simulink model "Gas_Exchange"  (Simulink 7.0)
settings: Solver=ode45  StartTime=0.0  StopTime=10.0  RelTol=1e-3
values from neighbouring files (symbols this model uses):
  a1 = 0.3836    [Dissociation_Spencer_IC.m]    (also in Gas_Exchange_IC.m; Respiratory_IC.m)
  a2 = 1.819    [Dissociation_Spencer_IC.m]    (also in Gas_Exchange_IC.m; Respiratory_IC.m)
  alpha1 = 0.02598    [Dissociation_Spencer_IC.m]    (also in Gas_Exchange_IC.m; Respiratory_IC.m)
  alpha2 = 0.05591    [Dissociation_Spencer_IC.m]    (also in Gas_Exchange_IC.m; Respiratory_IC.m)
  beta1 = 0.012275    [Dissociation_Spencer_IC.m]    (also in Gas_Exchange_IC.m; Respiratory_IC.m)
  beta2 = 0.03255    [Dissociation_Spencer_IC.m]    (also in Gas_Exchange_IC.m; Respiratory_IC.m)
  C1 = 9    [Dissociation_Spencer_IC.m]    (also in Gas_Exchange_IC.m; Respiratory_IC.m)
  C2 = 87.00    (= 87)    [Dissociation_Spencer_IC.m]    (also in Gas_Exchange_IC.m; Respiratory_IC.m)
  CvCO2IC = 0.5116    [Body_Khoo_IC.m]    (also in Gas_Exchange_IC.m; Respiratory_IC.m = 0.5247)
  CvO2IC = 0.1672    [Body_Khoo_IC.m]    (also in Gas_Exchange_IC.m; Respiratory_IC.m = 0.1639)
  Dead1CO2IC = 0.1020    (= 0.102)    [Dead_Space_Khoo_IC.m]    (also in Gas_Exchange_IC.m; Respiratory_IC.m = 39.5616)
  Dead1O2IC = 149.8824    [Dead_Space_Khoo_IC.m]    (also in Gas_Exchange_IC.m; Respiratory_IC.m = 104.3637)
  Dead2CO2IC = 0.5274    [Dead_Space_Khoo_IC.m]    (also in Gas_Exchange_IC.m; Respiratory_IC.m = 39.6736)
  Dead2O2IC = 149.3923    [Dead_Space_Khoo_IC.m]    (also in Gas_Exchange_IC.m; Respiratory_IC.m = 104.2258)
  Dead3CO2IC = 2.2996    [Dead_Space_Khoo_IC.m]    (also in Gas_Exchange_IC.m; Respiratory_IC.m = 39.8127)
  Dead3O2IC = 147.3503    [Dead_Space_Khoo_IC.m]    (also in Gas_Exchange_IC.m; Respiratory_IC.m = 104.0505)
  Dead4CO2IC = 8.2293    [Dead_Space_Khoo_IC.m]    (also in Gas_Exchange_IC.m; Respiratory_IC.m = 40.0061)
  Dead4O2IC = 140.5179    [Dead_Space_Khoo_IC.m]    (also in Gas_Exchange_IC.m; Respiratory_IC.m = 103.8005)
  Dead5CO2IC = 22.0757    [Dead_Space_Khoo_IC.m]    (also in Gas_Exchange_IC.m; Respiratory_IC.m = 40.3359)
  Dead5O2IC = 124.5641    [Dead_Space_Khoo_IC.m]    (also in Gas_Exchange_IC.m; Respiratory_IC.m = 103.3579)
  h = 0.0183    [Brain_Khoo_IC.m]    (also in Gas_Exchange_IC.m; Respiratory_IC.m)
  K1 = 13    [Dissociation_Spencer_IC.m]    (also in Gas_Exchange_IC.m; Respiratory_IC.m)
  K2 = 194.4    [Dissociation_Spencer_IC.m]    (also in Gas_Exchange_IC.m; Respiratory_IC.m)
  MRbCO2 = 0.0517    [Brain_Khoo_IC.m]    (also in Gas_Exchange_IC.m; Respiratory_IC.m)
  MRCO2 = 0.0033    [Body_Khoo_IC.m]    (also in Gas_Exchange_IC.m; Respiratory_IC.m)
  MRO2 = 0.0038    [Body_Khoo_IC.m]    (also in Gas_Exchange_IC.m; Respiratory_IC.m)
  PACO2_delayIC = 39.6041    [Cardio_Mix_Lange_IC.m]    (also in Gas_Exchange_IC.m; Respiratory_IC.m = 40.4448)
  PaCO2firstIC = 0.2150    (= 0.215)    [Cardio_Mix_Lange_IC.m]    (also in Gas_Exchange_IC.m; Respiratory_IC.m = -0.2465)
  PACO2IC = 37.1484    [Gas_Exchange_IC.m]    (also in Lungs_Khoo_IC.m; Respiratory_IC.m = 40.9432)
  PaCO2secondIC = 38.4577    [Cardio_Mix_Lange_IC.m]    (also in Gas_Exchange_IC.m; Respiratory_IC.m = 40.3928)
  PAO2_delayIC = 103.8436    [Cardio_Mix_Lange_IC.m]    (also in Gas_Exchange_IC.m; Respiratory_IC.m = 103.1223)
  PaO2firstIC = -0.2838    [Cardio_Mix_Lange_IC.m]    (also in Gas_Exchange_IC.m; Respiratory_IC.m = 0.3557)
  PAO2IC = 107.1983    [Gas_Exchange_IC.m]    (also in Lungs_Khoo_IC.m; Respiratory_IC.m = 102.5153)
  PaO2secondIC = 105.4828    [Cardio_Mix_Lange_IC.m]    (also in Gas_Exchange_IC.m; Respiratory_IC.m = 103.1435)
  PbCO2IC = 48.2858    [Brain_Khoo_IC.m]    (also in Gas_Exchange_IC.m; Respiratory_IC.m = 48.5383)
  PICO2 = 0    [Dead_Space_Khoo_IC.m]    (also in Gas_Exchange_IC.m; Respiratory_IC.m)
  PICO2_change = 0    [Respiratory_IC.m]
  PIO2 = 150    [Dead_Space_Khoo_IC.m]    (also in Gas_Exchange_IC.m; Respiratory_IC.m)
  PIO2_change = -90    [Mech_vent_test.m]    (also in Respiratory_IC.m = 0)
  QdBo = 0.8333    [Brain_Khoo_IC.m]    (also in Gas_Exchange_IC.m; Respiratory_IC.m)
  SbCO2 = 0.3600    (= 0.36)    [Brain_Khoo_IC.m]    (also in Gas_Exchange_IC.m; Respiratory_IC.m)
  SCO2 = 0.0043    [Brain_Khoo_IC.m]    (also in Gas_Exchange_IC.m; Respiratory_IC.m)
  T1 = 1    [Cardio_Mix_Lange_IC.m]    (also in Gas_Exchange_IC.m; Respiratory_IC.m)
  T2 = 2    [Cardio_Mix_Lange_IC.m]    (also in Gas_Exchange_IC.m; Respiratory_IC.m)
  t_CO2_duration = 0    [Respiratory_IC.m]
  t_CO2_start = 0    [Respiratory_IC.m]
  t_O2_duration = 0    [Mech_vent_test.m]    (also in Respiratory_IC.m)
  t_O2_start = 0    [Mech_vent_test.m]    (also in Respiratory_IC.m)
  Vdead1 = 0.03    [Dead_Space_Khoo_IC.m]    (also in Gas_Exchange_IC.m; Respiratory_IC.m)
  Vdead2 = 0.03    [Dead_Space_Khoo_IC.m]    (also in Gas_Exchange_IC.m; Respiratory_IC.m)
  Vdead3 = 0.03    [Dead_Space_Khoo_IC.m]    (also in Gas_Exchange_IC.m; Respiratory_IC.m)
  Vdead4 = 0.03    [Dead_Space_Khoo_IC.m]    (also in Gas_Exchange_IC.m; Respiratory_IC.m)
  Vdead5 = 0.03    [Dead_Space_Khoo_IC.m]    (also in Gas_Exchange_IC.m; Respiratory_IC.m)
  VTCO2 = 15    [Body_Khoo_IC.m]    (also in Gas_Exchange_IC.m; Respiratory_IC.m)
  VTO2 = 6    [Body_Khoo_IC.m]    (also in Gas_Exchange_IC.m; Respiratory_IC.m)
  Z = 0.0227    [Dissociation_Spencer_IC.m]    (also in Gas_Exchange_IC.m; Respiratory_IC.m)
settings Model: Creator=CLM  LastModifiedBy=CLM
settings OptimizationCC: BlockReduction=off  BooleanDataType=off
settings DebuggingCC: SaveWithParameterizedLinksMsg=none  SignalResolutionControl=TryResolveAllWithWarning  SolverPrmCheckMsg=none  MultiTaskDSMMsg=warning  MultiTaskCondExecSysMsg=none  StrictBusMsg=None
settings HardwareCC: TargetUnknown=on
settings RTWCC: IncludeERTFirstTime=on
settings GRTTargetCC: TargetFcnLib=ansi_tfl_tmw.mat

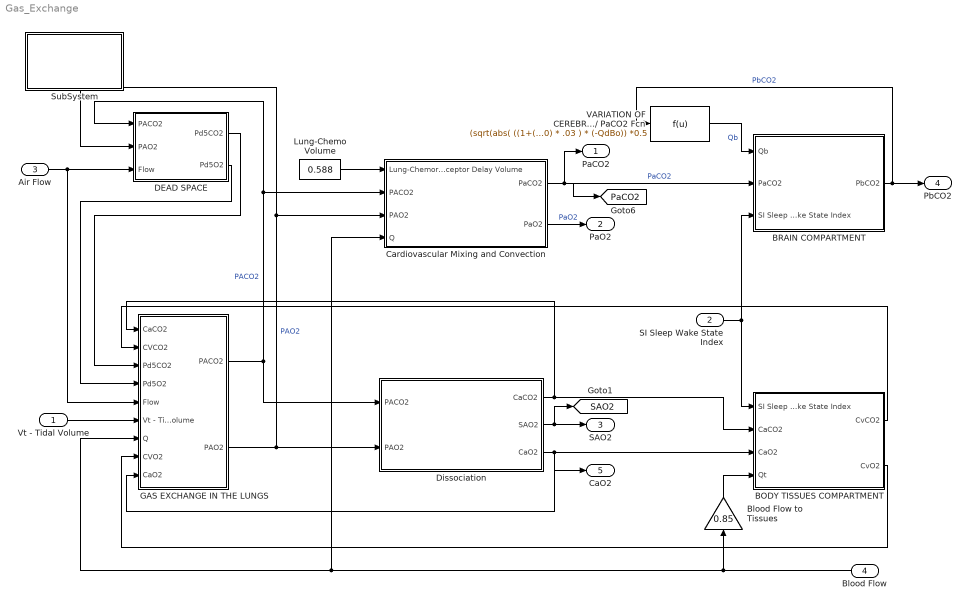
== system Gas_Exchange ==
  Vt - Tidal Volume : Inport  OutDataType=sfix(16)  OutScaling=2^0
  SI Sleep Wake State Index : Inport  Port=2  OutDataType=sfix(16)  OutScaling=2^0
  Air Flow : Inport  Port=3  OutDataType=sfix(16)  OutScaling=2^0
  Blood Flow : Inport  Orientation=left  Port=4  OutDataType=sfix(16)  OutScaling=2^0
  BODY TISSUES COMPARTMENT : Subsystem
  BRAIN COMPARTMENT : Subsystem
  Blood Flow to Tissues : Gain  Orientation=up  Gain=0.85  ParameterDataType=sfix(16)  ParameterScaling=2^0  OutDataType=sfix(16)  OutScaling=2^0  SaturateOnIntegerOverflow=on
  Cardiovascular Mixing and Convection : Subsystem
  DEAD SPACE : Subsystem
  Dissociation : Subsystem
  GAS EXCHANGE IN THE LUNGS : Subsystem
  Lung-Chemo Volume : Constant  Value=0.588  OutDataType=sfix(16)  OutScaling=2^0
  SubSystem : Subsystem
      settings: OpenFcn=Gas_Exchange_IC
      mask Display: disp('"double click here"\n to load \nGas_Exchange \ninitial values');
  VARIATION OF CEREBRAL BLOOD FLOW W/ PaCO2 Fcn : Fcn  Expr=(sqrt(abs( ((1+(u - 40) * .03 ) * (-QdBo))^2 - ( MRbCO2-h) * 4*0.03*QdBo/SCO2 ) )- (1+(u - 40) * .03 ) * (-QdBo)) *0.5
  PaCO2 : Outport  OutDataType=sfix(16)  OutScaling=2^0
  PaO2 : Outport  Port=2  OutDataType=sfix(16)  OutScaling=2^0
  SAO2 : Outport  Port=3  OutDataType=sfix(16)  OutScaling=2^0
  PbCO2 : Outport  Port=4  OutDataType=sfix(16)  OutScaling=2^0
  CaO2 : Outport  Port=5  OutDataType=sfix(16)  OutScaling=2^0
  tag scope: PaCO2=global, SAO2=global
  wires:
  SI Sleep Wake State Index/1 -> BODY TISSUES COMPARTMENT/1(SI Sleep Wake State Index), BRAIN COMPARTMENT/3(SI Sleep Wake State Index)
  Cardiovascular Mixing and Convection/1(PaCO2) -> PaCO2/1, BRAIN COMPARTMENT/2(PaCO2), [PaCO2]  "PaCO2"
  BRAIN COMPARTMENT/1(PbCO2) -> PbCO2/1, VARIATION OF CEREBRAL BLOOD FLOW W/ PaCO2 Fcn/1  "PbCO2"
  DEAD SPACE/1(Pd5CO2) -> GAS EXCHANGE IN THE LUNGS/3(Pd5CO2)
  DEAD SPACE/2(Pd5O2) -> GAS EXCHANGE IN THE LUNGS/4(Pd5O2)
  GAS EXCHANGE IN THE LUNGS/2(PAO2) -> DEAD SPACE/2(PAO2), Cardiovascular Mixing and Convection/3(PAO2), Dissociation/2(PAO2)  "PAO2"
  Vt - Tidal Volume/1 -> GAS EXCHANGE IN THE LUNGS/6(Vt - Tidal Volume)
  Air Flow/1 -> DEAD SPACE/3(Flow), GAS EXCHANGE IN THE LUNGS/5(Flow)
  VARIATION OF CEREBRAL BLOOD FLOW W/ PaCO2 Fcn/1 -> BRAIN COMPARTMENT/1(Qb)  "Qb"
  GAS EXCHANGE IN THE LUNGS/1(PACO2) -> DEAD SPACE/1(PACO2), Cardiovascular Mixing and Convection/2(PACO2), Dissociation/1(PACO2)  "PACO2"
  Lung-Chemo Volume/1 -> Cardiovascular Mixing and Convection/1(Lung-Chemoreceptor Delay Volume)
  Blood Flow/1 -> Blood Flow to Tissues/1, GAS EXCHANGE IN THE LUNGS/7("Q "), Cardiovascular Mixing and Convection/4(Q)
  Cardiovascular Mixing and Convection/2(PaO2) -> PaO2/1  "PaO2"
  Blood Flow to Tissues/1 -> BODY TISSUES COMPARTMENT/4("Qt ")
  Dissociation/1(CaCO2) -> GAS EXCHANGE IN THE LUNGS/1(CaCO2), BODY TISSUES COMPARTMENT/2(CaCO2)
  Dissociation/3(CaO2) -> GAS EXCHANGE IN THE LUNGS/9(CaO2), CaO2/1, BODY TISSUES COMPARTMENT/3(CaO2)
  Dissociation/2(SAO2) -> [SAO2], SAO2/1
  BODY TISSUES COMPARTMENT/1(CvCO2) -> GAS EXCHANGE IN THE LUNGS/2(CVCO2)
  BODY TISSUES COMPARTMENT/2(CvO2) -> GAS EXCHANGE IN THE LUNGS/8(CVO2)

== system Gas_Exchange/BODY TISSUES COMPARTMENT ==
  SI Sleep Wake State Index : Inport  Orientation=left  OutDataType=sfix(16)  OutScaling=2^0
  CaCO2 : Inport  Orientation=left  Port=2  OutDataType=sfix(16)  OutScaling=2^0
  CaO2 : Inport  Orientation=left  Port=3  OutDataType=sfix(16)  OutScaling=2^0
  "Qt " : Inport  Orientation=left  Port=4  OutDataType=sfix(16)  OutScaling=2^0
  Body Tissues Compartment for CO2 : Subsystem  Orientation=left
  Body Tissues Compartment for O2 : Subsystem  Orientation=left
  CvCO2 : Outport  Orientation=left  OutDataType=sfix(16)  OutScaling=2^0
  CvO2 : Outport  Orientation=left  Port=2  OutDataType=sfix(16)  OutScaling=2^0
  wires:
  SI Sleep Wake State Index/1 -> Body Tissues Compartment for CO2/3(SI Sleep Wake State Index), Body Tissues Compartment for O2/2(SI Sleep Wake State Index)
  CaCO2/1 -> Body Tissues Compartment for CO2/1(CaCO2)
  CaO2/1 -> Body Tissues Compartment for O2/3(CaO2)
  Body Tissues Compartment for CO2/1(CvCO2) -> CvCO2/1
  Body Tissues Compartment for O2/1(CVO2) -> CvO2/1
  "Qt "/1 -> Body Tissues Compartment for O2/1(Qt), Body Tissues Compartment for CO2/2(Qt)

== system Gas_Exchange/BRAIN COMPARTMENT ==
  Qb : Inport  OutDataType=sfix(16)  OutScaling=2^0
  PaCO2 : Inport  Port=2  OutDataType=sfix(16)  OutScaling=2^0
  SI Sleep Wake State Index : Inport  Port=3  OutDataType=sfix(16)  OutScaling=2^0
  Fcn : Fcn  Expr=MRbCO2*(0.375*(1-0.4*u)+0.625)
  Fcn -5 blocks : Fcn  Expr=(u(1) + ( u(2) * u(3)) *SCO2- h ) /SbCO2
  Integrator : Integrator  InitialCondition=PbCO2IC
  Mux : Mux  Inputs=3
  sum : Sum  Inputs=+-  OutDataType=sfix(16)  OutScaling=2^0  SaturateOnIntegerOverflow=on  InputSameDT=on
  PbCO2 : Outport  OutDataType=sfix(16)  OutScaling=2^0
  tag scope: PbCO2IC=global
  wires:
  Fcn -5 blocks/1 -> Integrator/1
  PaCO2/1 -> sum/1
  Integrator/1 -> sum/2, [PbCO2IC], PbCO2/1
  SI Sleep Wake State Index/1 -> Fcn/1
  Mux/1 -> Fcn -5 blocks/1
  Fcn/1 -> Mux/1
  Qb/1 -> Mux/2
  sum/1 -> Mux/3

== system Gas_Exchange/Cardiovascular Mixing and Convection ==
  Lung-Chemoreceptor Delay Volume : Inport  OutDataType=sfix(16)  OutScaling=2^0
  PACO2 : Inport  Port=2  OutDataType=sfix(16)  OutScaling=2^0
  PAO2 : Inport  Port=3  OutDataType=sfix(16)  OutScaling=2^0
  Q : Inport  Port=4  OutDataType=sfix(16)  OutScaling=2^0
  CO2 Cardiovascular Mixing and Convection Effects : Subsystem
  O2 Cardiovascular Mixing and Convection Effects : Subsystem
  PaCO2 : Outport  OutDataType=sfix(16)  OutScaling=2^0
  PaO2 : Outport  Port=2  OutDataType=sfix(16)  OutScaling=2^0
  wires:
  CO2 Cardiovascular Mixing and Convection Effects/1(PaCO2) -> PaCO2/1
  PACO2/1 -> CO2 Cardiovascular Mixing and Convection Effects/1(PACO2)
  Q/1 -> CO2 Cardiovascular Mixing and Convection Effects/2(Q), O2 Cardiovascular Mixing and Convection Effects/1(Q)
  Lung-Chemoreceptor Delay Volume/1 -> CO2 Cardiovascular Mixing and Convection Effects/3(Lung-Chemoreceptor Delay Volume), O2 Cardiovascular Mixing and Convection Effects/3(Lung-Chemoreceptor Delay Volume)
  O2 Cardiovascular Mixing and Convection Effects/1(PaO2) -> PaO2/1
  PAO2/1 -> O2 Cardiovascular Mixing and Convection Effects/2(PAO2)

== system Gas_Exchange/DEAD SPACE ==
  PACO2 : Inport  OutDataType=sfix(16)  OutScaling=2^0
  PAO2 : Inport  Port=2  OutDataType=sfix(16)  OutScaling=2^0
  Flow : Inport  Port=3  OutDataType=sfix(16)  OutScaling=2^0
  CO2 DEAD SPACE : Subsystem
  O2 DEAD SPACE : Subsystem
  Pd5CO2 : Outport  OutDataType=sfix(16)  OutScaling=2^0
  Pd5O2 : Outport  Port=2  OutDataType=sfix(16)  OutScaling=2^0
  wires:
  PACO2/1 -> CO2 DEAD SPACE/1(PACO2)
  PAO2/1 -> O2 DEAD SPACE/2(PAO2)
  CO2 DEAD SPACE/1(Pd5CO2) -> Pd5CO2/1
  O2 DEAD SPACE/1(Pd5O2) -> Pd5O2/1
  Flow/1 -> CO2 DEAD SPACE/2(Flow), O2 DEAD SPACE/1(Flow)

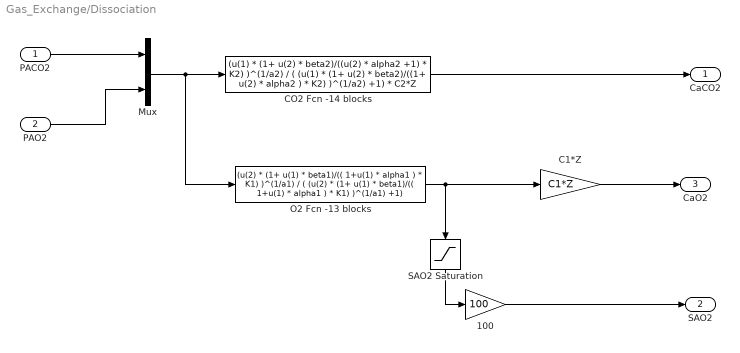
== system Gas_Exchange/Dissociation ==
  PACO2 : Inport  OutDataType=sfix(16)  OutScaling=2^0
  PAO2 : Inport  Port=2  OutDataType=sfix(16)  OutScaling=2^0
  100 : Gain  Gain=100  ParameterDataType=sfix(16)  ParameterScaling=2^0  OutDataType=sfix(16)  OutScaling=2^0  SaturateOnIntegerOverflow=on
  C1*Z : Gain  Gain=C1*Z  ParameterDataType=sfix(16)  ParameterScaling=2^0  OutDataType=sfix(16)  OutScaling=2^0  SaturateOnIntegerOverflow=on
  CO2 Fcn -14 blocks : Fcn  Expr="(u(1) * (1+ u(2) * beta2)/((u(2) * alpha2 +1) * K2) )^(1/a2) / ( (u(1) * (1+ u(2) * beta2)/((1+ u(2) * alpha2 ) * K2) )^(1/a2)  +1) * C2*Z"
  Mux : Mux  Inputs=2
  O2 Fcn -13 blocks : Fcn  Expr="(u(2) * (1+ u(1) * beta1)/(( 1+u(1) * alpha1 ) * K1) )^(1/a1) / ( (u(2) * (1+ u(1) * beta1)/(( 1+u(1) * alpha1 ) * K1) )^(1/a1)   +1)"
  SAO2 Saturation : Saturate  Orientation=down  UpperLimit=5  LowerLimit=-5
  CaCO2 : Outport  OutDataType=sfix(16)  OutScaling=2^0
  SAO2 : Outport  Port=2  OutDataType=sfix(16)  OutScaling=2^0
  CaO2 : Outport  Port=3  OutDataType=sfix(16)  OutScaling=2^0
  wires:
  CO2 Fcn -14 blocks/1 -> CaCO2/1
  C1*Z/1 -> CaO2/1
  O2 Fcn -13 blocks/1 -> C1*Z/1, SAO2 Saturation/1
  PACO2/1 -> Mux/1
  PAO2/1 -> Mux/2
  100/1 -> SAO2/1
  SAO2 Saturation/1 -> 100/1
  Mux/1 -> CO2 Fcn -14 blocks/1, O2 Fcn -13 blocks/1

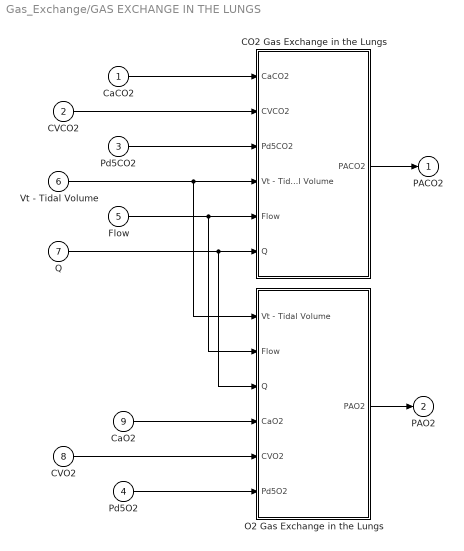
== system Gas_Exchange/GAS EXCHANGE IN THE LUNGS ==
  CaCO2 : Inport  OutDataType=sfix(16)  OutScaling=2^0
  CVCO2 : Inport  Port=2  OutDataType=sfix(16)  OutScaling=2^0
  Pd5CO2 : Inport  Port=3  OutDataType=sfix(16)  OutScaling=2^0
  Pd5O2 : Inport  Port=4  OutDataType=sfix(16)  OutScaling=2^0
  Flow : Inport  Port=5  OutDataType=sfix(16)  OutScaling=2^0
  Vt - Tidal Volume : Inport  Port=6  OutDataType=sfix(16)  OutScaling=2^0
  "Q " : Inport  Port=7  OutDataType=sfix(16)  OutScaling=2^0
  CVO2 : Inport  Port=8  OutDataType=sfix(16)  OutScaling=2^0
  CaO2 : Inport  Port=9  OutDataType=sfix(16)  OutScaling=2^0
  CO2 Gas Exchange in the Lungs : Subsystem
  O2 Gas Exchange in the Lungs : Subsystem
  PACO2 : Outport  OutDataType=sfix(16)  OutScaling=2^0
  PAO2 : Outport  Port=2  OutDataType=sfix(16)  OutScaling=2^0
  wires:
  CO2 Gas Exchange in the Lungs/1(PACO2) -> PACO2/1
  O2 Gas Exchange in the Lungs/1(PAO2) -> PAO2/1
  CaCO2/1 -> CO2 Gas Exchange in the Lungs/1(CaCO2)
  CVCO2/1 -> CO2 Gas Exchange in the Lungs/2(CVCO2)
  Pd5CO2/1 -> CO2 Gas Exchange in the Lungs/3(Pd5CO2)
  Vt - Tidal Volume/1 -> O2 Gas Exchange in the Lungs/1(Vt - Tidal Volume), CO2 Gas Exchange in the Lungs/4(Vt - Tidal Volume)
  Flow/1 -> O2 Gas Exchange in the Lungs/2(Flow), CO2 Gas Exchange in the Lungs/5(Flow)
  "Q "/1 -> O2 Gas Exchange in the Lungs/3(Q), CO2 Gas Exchange in the Lungs/6("Q ")
  CaO2/1 -> O2 Gas Exchange in the Lungs/4(CaO2)
  CVO2/1 -> O2 Gas Exchange in the Lungs/5(CVO2)
  Pd5O2/1 -> O2 Gas Exchange in the Lungs/6(Pd5O2)

== system Gas_Exchange/SubSystem ==

== system Gas_Exchange/BODY TISSUES COMPARTMENT/Body Tissues Compartment for CO2 ==
  CaCO2 : Inport  OutDataType=sfix(16)  OutScaling=2^0
  Qt : Inport  Port=2  OutDataType=sfix(16)  OutScaling=2^0
  SI Sleep Wake State Index : Inport  Port=3  OutDataType=sfix(16)  OutScaling=2^0
  Fcn : Fcn  Expr=MRCO2*(0.375*(1-0.4*u)+0.625)
  Fcn -5 blocks : Fcn  Expr=( u(1) + ( u(2) * u(3)) ) /VTCO2
  Integrator : Integrator  InitialCondition=CvCO2IC
  Mux : Mux  Inputs=3
  Sum1 : Sum  Inputs=+-  OutDataType=sfix(16)  OutScaling=2^0  SaturateOnIntegerOverflow=on  InputSameDT=on
  CvCO2 : Outport  OutDataType=sfix(16)  OutScaling=2^0
  tag scope: CvCO2IC=global
  wires:
  SI Sleep Wake State Index/1 -> Fcn/1
  CaCO2/1 -> Sum1/1
  Fcn -5 blocks/1 -> Integrator/1
  Integrator/1 -> [CvCO2IC], Sum1/2, CvCO2/1
  Mux/1 -> Fcn -5 blocks/1
  Fcn/1 -> Mux/1
  Qt/1 -> Mux/2
  Sum1/1 -> Mux/3

== system Gas_Exchange/BODY TISSUES COMPARTMENT/Body Tissues Compartment for O2 ==
  Qt : Inport  OutDataType=sfix(16)  OutScaling=2^0
  SI Sleep Wake State Index : Inport  Port=2  OutDataType=sfix(16)  OutScaling=2^0
  CaO2 : Inport  Port=3  OutDataType=sfix(16)  OutScaling=2^0
  Fcn : Fcn  Expr=MRO2*(0.375*(1-0.4*u)+0.625)
  Fcn -5 blocks : Fcn  Expr=( -u(1) + ( u(2) * u(3)) ) /VTO2
  Integrator : Integrator  InitialCondition=CvO2IC
  Mux : Mux  Inputs=3
  Sum1 : Sum  Inputs=+-  OutDataType=sfix(16)  OutScaling=2^0  SaturateOnIntegerOverflow=on  InputSameDT=on
  CVO2 : Outport  OutDataType=sfix(16)  OutScaling=2^0
  tag scope: CvO2IC=global
  wires:
  SI Sleep Wake State Index/1 -> Fcn/1
  Qt/1 -> Mux/2
  Sum1/1 -> Mux/3
  CaO2/1 -> Sum1/1
  Fcn -5 blocks/1 -> Integrator/1
  Integrator/1 -> [CvO2IC], Sum1/2, CVO2/1
  Mux/1 -> Fcn -5 blocks/1
  Fcn/1 -> Mux/1

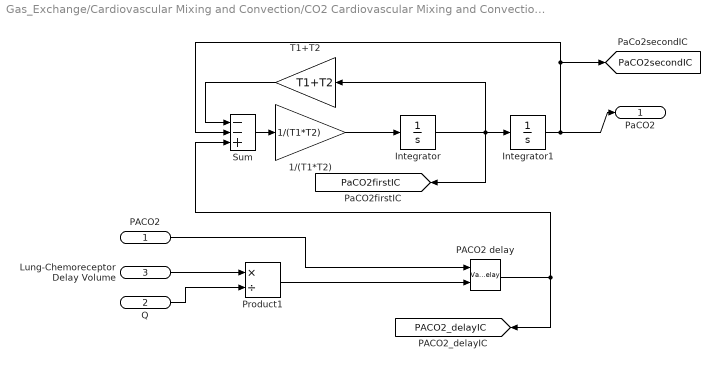
== system Gas_Exchange/Cardiovascular Mixing and Convection/CO2 Cardiovascular Mixing and Convection Effects ==
  PACO2 : Inport  OutDataType=sfix(16)  OutScaling=2^0
  Q : Inport  Port=2  OutDataType=sfix(16)  OutScaling=2^0
  Lung-Chemoreceptor Delay Volume : Inport  Port=3  OutDataType=sfix(16)  OutScaling=2^0
  1/(T1*T2) : Gain  Gain=1/(T1*T2)  ParameterDataType=sfix(16)  ParameterScaling=2^0  OutDataType=sfix(16)  OutScaling=2^0  SaturateOnIntegerOverflow=on
  Integrator : Integrator  InitialCondition=PaCO2firstIC
  Integrator1 : Integrator  InitialCondition=PaCO2secondIC
  PACO2 delay : VariableTransportDelay  MaximumDelay=100  InitialOutput=PACO2_delayIC  MaximumPoints=22528
  Product1 : Product  Inputs=*/  OutDataType=sfix(16)  OutScaling=2^0  SaturateOnIntegerOverflow=on  InputSameDT=on
  Sum : Sum  Inputs=--+  OutDataType=sfix(16)  OutScaling=2^0  SaturateOnIntegerOverflow=on  InputSameDT=on
  T1+T2 : Gain  Orientation=left  Gain=T1+T2  ParameterDataType=sfix(16)  ParameterScaling=2^0  OutDataType=sfix(16)  OutScaling=2^0  SaturateOnIntegerOverflow=on
  PaCO2 : Outport  OutDataType=sfix(16)  OutScaling=2^0
  tag scope: PACO2_delayIC=global, PaCO2firstIC=global, PaCO2secondIC=global
  wires:
  T1+T2/1 -> Sum/1
  Integrator/1 -> T1+T2/1, Integrator1/1, [PaCO2firstIC]
  Sum/1 -> 1/(T1*T2)/1
  1/(T1*T2)/1 -> Integrator/1
  Integrator1/1 -> Sum/2, [PaCO2secondIC], PaCO2/1
  PACO2/1 -> PACO2 delay/1
  PACO2 delay/1 -> [PACO2_delayIC], Sum/3
  Product1/1 -> PACO2 delay/2
  Lung-Chemoreceptor Delay Volume/1 -> Product1/1
  Q/1 -> Product1/2

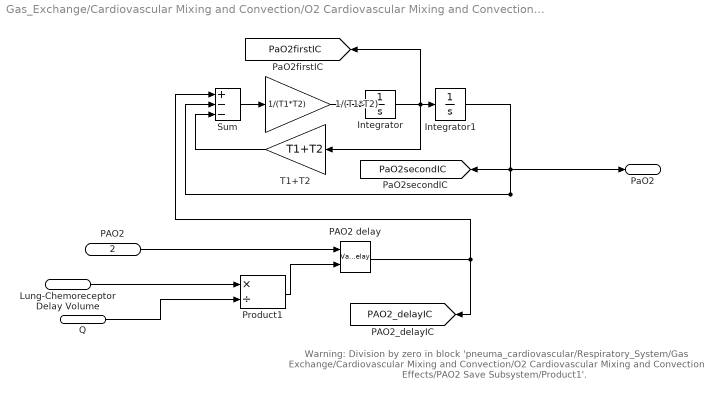
== system Gas_Exchange/Cardiovascular Mixing and Convection/O2 Cardiovascular Mixing and Convection Effects ==
  note: Warning: Division by zero in block 'pneuma_cardiovascular/Respiratory_System/Gas Exchange/Cardiovascular Mixing and Convection/O2 Cardiovascular Mixing and Convection Effects/PAO2 Save Subsystem/Product1'.
  Q : Inport  OutDataType=sfix(16)  OutScaling=2^0
  PAO2 : Inport  Port=2  OutDataType=sfix(16)  OutScaling=2^0
  Lung-Chemoreceptor Delay Volume : Inport  Port=3  OutDataType=sfix(16)  OutScaling=2^0
  1/(T1*T2) : Gain  Gain=1/(T1*T2)  ParameterDataType=sfix(16)  ParameterScaling=2^0  OutDataType=sfix(16)  OutScaling=2^0  SaturateOnIntegerOverflow=on
  Integrator : Integrator  InitialCondition=PaO2firstIC
  Integrator1 : Integrator  InitialCondition=PaO2secondIC
  PAO2 delay : VariableTransportDelay  MaximumDelay=100  InitialOutput=PAO2_delayIC  MaximumPoints=22528
  Product1 : Product  Inputs=*/  OutDataType=sfix(16)  OutScaling=2^0  SaturateOnIntegerOverflow=on  InputSameDT=on
  Sum : Sum  Inputs=+--  OutDataType=sfix(16)  OutScaling=2^0  SaturateOnIntegerOverflow=on  InputSameDT=on
  T1+T2 : Gain  Orientation=left  Gain=T1+T2  ParameterDataType=sfix(16)  ParameterScaling=2^0  OutDataType=sfix(16)  OutScaling=2^0  SaturateOnIntegerOverflow=on
  PaO2 : Outport  OutDataType=sfix(16)  OutScaling=2^0
  tag scope: PAO2_delayIC=global, PaO2firstIC=global, PaO2secondIC=global
  wires:
  1/(T1*T2)/1 -> Integrator/1
  Sum/1 -> 1/(T1*T2)/1
  Integrator/1 -> Integrator1/1, T1+T2/1, [PaO2firstIC]
  Integrator1/1 -> [PaO2secondIC], Sum/2, PaO2/1
  T1+T2/1 -> Sum/3
  Product1/1 -> PAO2 delay/2
  PAO2/1 -> PAO2 delay/1
  PAO2 delay/1 -> [PAO2_delayIC], Sum/1
  Lung-Chemoreceptor Delay Volume/1 -> Product1/1
  Q/1 -> Product1/2

== system Gas_Exchange/DEAD SPACE/CO2 DEAD SPACE ==
  PACO2 : Inport  OutDataType=sfix(16)  OutScaling=2^0
  Flow : Inport  Port=2  OutDataType=sfix(16)  OutScaling=2^0
  CO2 Partial Pressure : Subsystem  mask{begin_time=t_CO2_start, end_time=t_CO2_start+t_CO2_duration, init_value=PICO2, final_value=PICO2+PICO2_change}
      mask prompts: begin_time "pulse begin"; end_time "pulse end"; init_value "initial value"; final_value "final value"
      mask Display: disp('pulse')
  Pd(1)CO2 : Subsystem
  Pd(2)CO2 : Subsystem
  Pd(3)CO2 : Subsystem
  Pd(4)CO2 : Subsystem
  Pd(5)CO2 : Subsystem
  Pd5CO2 : Outport  OutDataType=sfix(16)  OutScaling=2^0
  wires:
  Pd(4)CO2/1(Pd(4)CO2) -> Pd(3)CO2/3(Pd(4)CO2), Pd(5)CO2/1(Pd(4)CO2)
  Pd(3)CO2/1(Pd(3)CO2) -> Pd(4)CO2/1(Pd(3)CO2), Pd(2)CO2/3(Pd(3)CO2)
  Pd(2)CO2/1(Pd(2)CO2) -> Pd(3)CO2/1(Pd(2)CO2), Pd(1)CO2/3(Pd(2)CO2)
  Pd(1)CO2/1(Pd(1)CO2) -> Pd(2)CO2/1(Pd(1)CO2)
  Flow/1 -> Pd(1)CO2/2(Flow), Pd(2)CO2/2(Flow), Pd(4)CO2/2(Flow), Pd(5)CO2/2(Flow), Pd(3)CO2/2(Flow)
  PACO2/1 -> Pd(5)CO2/3(PACO2)
  Pd(5)CO2/1(Pd(5)CO2) -> Pd5CO2/1, Pd(4)CO2/3(Pd(5)CO2)
  CO2 Partial Pressure/1(Out1) -> Pd(1)CO2/1(PICO2)

== system Gas_Exchange/DEAD SPACE/O2 DEAD SPACE ==
  Flow : Inport  OutDataType=sfix(16)  OutScaling=2^0
  PAO2 : Inport  Port=2  OutDataType=sfix(16)  OutScaling=2^0
  O2 Partial Pressure : Subsystem  mask{begin_time=t_O2_start, end_time=t_O2_start+t_O2_duration, init_value=PIO2, final_value=PIO2+PIO2_change}
      mask prompts: begin_time "pulse begin"; end_time "pulse end"; init_value "initial value"; final_value "final value"
      mask Display: disp('pulse')
  Pd(1)O2 : Subsystem
  Pd(2)O2 : Subsystem
  Pd(3)O2 : Subsystem
  Pd(4)O2 : Subsystem
  Pd(5)O2 : Subsystem
  Pd5O2 : Outport  OutDataType=sfix(16)  OutScaling=2^0
  wires:
  Pd(4)O2/1(Pd(4)O2) -> Pd(3)O2/3(Pd(4)O2), Pd(5)O2/1(Pd(4)O2)
  Pd(3)O2/1(Pd(3)O2) -> Pd(4)O2/1(Pd(3)O2), Pd(2)O2/3(Pd(3)O2)
  Pd(2)O2/1(Pd(2)O2) -> Pd(3)O2/1(Pd(2)O2), Pd(1)O2/3(Pd(2)O2)
  Pd(1)O2/1(Pd(1)O2) -> Pd(2)O2/1(Pd(1)O2)
  PAO2/1 -> Pd(5)O2/3(PAO2)
  Flow/1 -> Pd(4)O2/2(Flow), Pd(5)O2/2(Flow), Pd(2)O2/2(Flow), Pd(1)O2/2(Flow), Pd(3)O2/2(Flow)
  Pd(5)O2/1(Pd(5)O2) -> Pd5O2/1, Pd(4)O2/3(Pd(5)O2)
  O2 Partial Pressure/1(Out1) -> Pd(1)O2/1(PIO2)

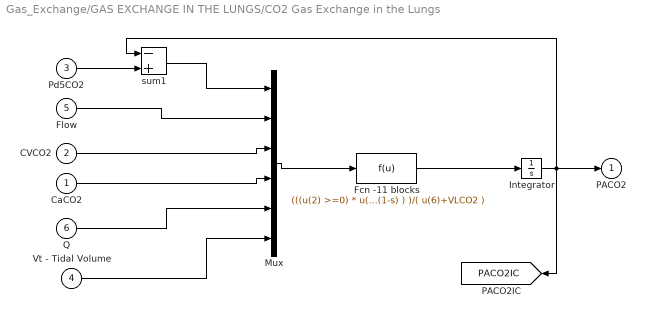
== system Gas_Exchange/GAS EXCHANGE IN THE LUNGS/CO2 Gas Exchange in the Lungs ==
  CaCO2 : Inport  OutDataType=sfix(16)  OutScaling=2^0
  CVCO2 : Inport  Port=2  OutDataType=sfix(16)  OutScaling=2^0
  Pd5CO2 : Inport  Port=3  OutDataType=sfix(16)  OutScaling=2^0
  Vt - Tidal Volume : Inport  Port=4  OutDataType=sfix(16)  OutScaling=2^0
  Flow : Inport  Port=5  OutDataType=sfix(16)  OutScaling=2^0
  "Q " : Inport  Port=6  OutDataType=sfix(16)  OutScaling=2^0
  Fcn -11 blocks : Fcn  Expr=(((u(2) >=0) * u(2) * u(1) + (u(2) <0) * 0 ) + (u(3) - u(4)) *u(5) * ( lambda*(1-s) ) )/( u(6)+VLCO2 )
  Integrator : Integrator  InitialCondition=PACO2IC
  Mux : Mux  Inputs=6
  sum1 : Sum  Inputs=-+  OutDataType=sfix(16)  OutScaling=2^0  SaturateOnIntegerOverflow=on  InputSameDT=on
  PACO2 : Outport  OutDataType=sfix(16)  OutScaling=2^0
  tag scope: PACO2IC=global
  wires:
  "Q "/1 -> Mux/5
  CVCO2/1 -> Mux/3
  CaCO2/1 -> Mux/4
  Fcn -11 blocks/1 -> Integrator/1
  Integrator/1 -> [PACO2IC], PACO2/1, sum1/1
  Pd5CO2/1 -> sum1/2
  Mux/1 -> Fcn -11 blocks/1
  sum1/1 -> Mux/1
  Flow/1 -> Mux/2
  Vt - Tidal Volume/1 -> Mux/6

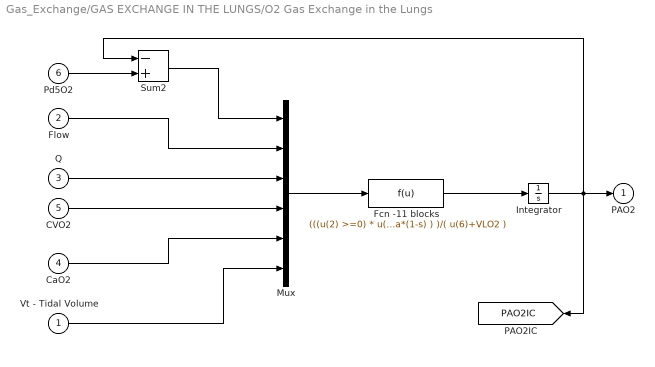
== system Gas_Exchange/GAS EXCHANGE IN THE LUNGS/O2 Gas Exchange in the Lungs ==
  Vt - Tidal Volume : Inport  OutDataType=sfix(16)  OutScaling=2^0
  Flow : Inport  Port=2  OutDataType=sfix(16)  OutScaling=2^0
  Q : Inport  Port=3  OutDataType=sfix(16)  OutScaling=2^0
  CaO2 : Inport  Port=4  OutDataType=sfix(16)  OutScaling=2^0
  CVO2 : Inport  Port=5  OutDataType=sfix(16)  OutScaling=2^0
  Pd5O2 : Inport  Port=6  OutDataType=sfix(16)  OutScaling=2^0
  Fcn -11 blocks : Fcn  Expr=(((u(2) >=0) * u(2) * u(1) + (u(2) <0) * 0 ) + (u(4) - u(5)) *u(3) * ( lambda*(1-s) ) )/( u(6)+VLO2 )
  Integrator : Integrator  InitialCondition=PAO2IC  LimitOutput=on  LowerSaturationLimit=0
  Mux : Mux  Inputs=6
  Sum2 : Sum  Inputs=-+  OutDataType=sfix(16)  OutScaling=2^0  SaturateOnIntegerOverflow=on  InputSameDT=on
  PAO2 : Outport  OutDataType=sfix(16)  OutScaling=2^0
  tag scope: PAO2IC=global
  wires:
  Integrator/1 -> PAO2/1, [PAO2IC], Sum2/1
  Fcn -11 blocks/1 -> Integrator/1
  Pd5O2/1 -> Sum2/2
  Mux/1 -> Fcn -11 blocks/1
  Sum2/1 -> Mux/1
  Flow/1 -> Mux/2
  Q/1 -> Mux/3
  CVO2/1 -> Mux/4
  CaO2/1 -> Mux/5
  Vt - Tidal Volume/1 -> Mux/6

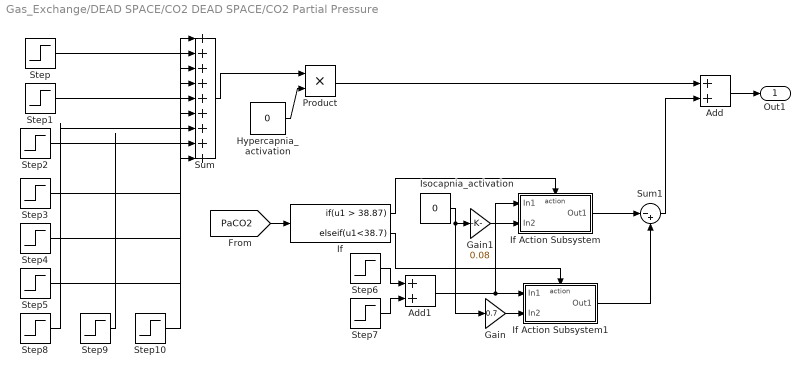
== system Gas_Exchange/DEAD SPACE/CO2 DEAD SPACE/CO2 Partial Pressure ==
  Add : Sum  OutDataType=sfix(16)  OutScaling=2^-10
  Add1 : Sum  OutDataType=sfix(16)  OutScaling=2^-10
  Gain : Gain  Gain=0.7  ParameterDataType=sfix(16)  ParameterScaling=2^0  OutDataType=sfix(16)  OutScaling=2^0
  Gain1 : Gain  Gain=0.08  ParameterDataType=sfix(16)  ParameterScaling=2^0  OutDataType=sfix(16)  OutScaling=2^0
  Hypercapnia_activation : Constant  Value=0  OutDataType=sfix(16)  OutScaling=2^0
  If : If  IfExpression=u1 > 38.87  ElseIfExpressions=u1<38.7  ShowElse=off
  If Action Subsystem : Subsystem  TreatAsAtomicUnit=on
  If Action Subsystem1 : Subsystem  TreatAsAtomicUnit=on
  Isocapnia_activation : Constant  Value=0  OutDataType=sfix(16)  OutScaling=2^0
  Product : Product  OutDataType=sfix(16)  OutScaling=2^0  RndMeth=Zero
  Step : Step  Time=begin_time  Before=init_value  After=final_value/8  SampleTime=0
  Step1 : Step  Time=end_time  After=init_value-final_value  SampleTime=0
  Step10 : Step  Time=begin_time+18  Before=init_value  After=final_value/8  SampleTime=0
  Step2 : Step  Time=begin_time+3  Before=init_value  After=final_value/8  SampleTime=0
  Step3 : Step  Time=begin_time+6  Before=init_value  After=final_value/8  SampleTime=0
  Step4 : Step  Time=begin_time+9  Before=init_value  After=final_value/8  SampleTime=0
  Step5 : Step  Time=begin_time+12  Before=init_value  After=final_value/8  SampleTime=0
  Step6 : Step  Time=begin_time  SampleTime=0
  Step7 : Step  Time=end_time  After=-1  SampleTime=0
  Step8 : Step  Time=begin_time+14  Before=init_value  After=final_value/8  SampleTime=0
  Step9 : Step  Time=begin_time+16  Before=init_value  After=final_value/8  SampleTime=0
  Sum : Sum  Inputs=|+++++++++  OutDataType=sfix(16)  OutScaling=2^0  SaturateOnIntegerOverflow=on  InputSameDT=on
  Sum1 : Sum  Inputs=|-+  OutDataType=sfix(16)  OutScaling=2^0
  Out1 : Outport  OutDataType=sfix(16)  OutScaling=2^0
  wires:
  [PaCO2] -> If/1
  Add/1 -> Out1/1
  Step6/1 -> Add1/1
  Step7/1 -> Add1/2
  Sum1/1 -> Add/2
  If/1 -> If Action Subsystem/Action
  If/2 -> If Action Subsystem1/Action
  Add1/1 -> If Action Subsystem1/1(In1), If Action Subsystem/1(In1)
  Isocapnia_activation/1 -> Gain1/1, Gain/1
  If Action Subsystem/1(Out1) -> Sum1/1
  If Action Subsystem1/1(Out1) -> Sum1/2
  Step/1 -> Sum/1
  Step1/1 -> Sum/2
  Step2/1 -> Sum/3
  Step3/1 -> Sum/4
  Step4/1 -> Sum/5
  Step5/1 -> Sum/6
  Sum/1 -> Product/1
  Hypercapnia_activation/1 -> Product/2
  Product/1 -> Add/1
  Step8/1 -> Sum/7
  Step9/1 -> Sum/8
  Step10/1 -> Sum/9
  Gain/1 -> If Action Subsystem1/2(In2)
  Gain1/1 -> If Action Subsystem/2(In2)

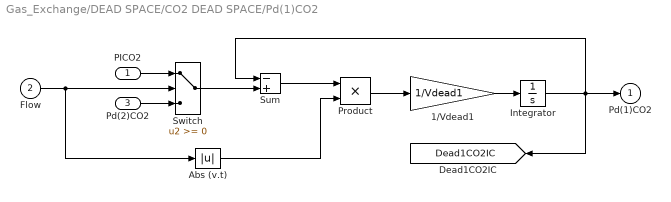
== system Gas_Exchange/DEAD SPACE/CO2 DEAD SPACE/Pd(1)CO2 ==
  PICO2 : Inport  OutDataType=sfix(16)  OutScaling=2^0
  Flow : Inport  Port=2  OutDataType=sfix(16)  OutScaling=2^0
  Pd(2)CO2 : Inport  Port=3  OutDataType=sfix(16)  OutScaling=2^0
  1/Vdead1 : Gain  Gain=1/Vdead1  ParameterDataType=sfix(16)  ParameterScaling=2^0  OutDataType=sfix(16)  OutScaling=2^0  SaturateOnIntegerOverflow=on
  Abs (v.t) : Abs  SaturateOnIntegerOverflow=on
  Integrator : Integrator  InitialCondition=Dead1CO2IC
  Product : Product  OutDataType=sfix(16)  OutScaling=2^0  SaturateOnIntegerOverflow=on  InputSameDT=on
  Sum : Sum  Inputs=-+  OutDataType=sfix(16)  OutScaling=2^0  SaturateOnIntegerOverflow=on  InputSameDT=on
  Switch : Switch  SaturateOnIntegerOverflow=on  InputSameDT=on
  Pd(1)CO2 : Outport  OutDataType=sfix(16)  OutScaling=2^0
  tag scope: Dead1CO2IC=global
  wires:
  Flow/1 -> Abs (v.t)/1, Switch/2
  Abs (v.t)/1 -> Product/2
  Switch/1 -> Sum/2
  Product/1 -> 1/Vdead1/1
  1/Vdead1/1 -> Integrator/1
  Integrator/1 -> [Dead1CO2IC], Pd(1)CO2/1, Sum/1
  Sum/1 -> Product/1
  PICO2/1 -> Switch/1
  Pd(2)CO2/1 -> Switch/3

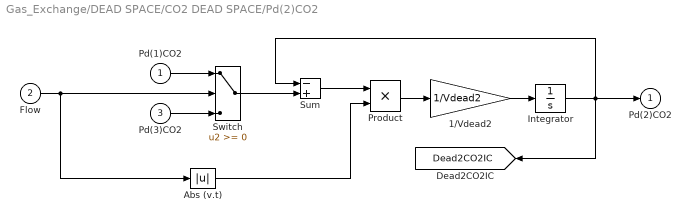
== system Gas_Exchange/DEAD SPACE/CO2 DEAD SPACE/Pd(2)CO2 ==
  Pd(1)CO2 : Inport  OutDataType=sfix(16)  OutScaling=2^0
  Flow : Inport  Port=2  OutDataType=sfix(16)  OutScaling=2^0
  Pd(3)CO2 : Inport  Port=3  OutDataType=sfix(16)  OutScaling=2^0
  1/Vdead2 : Gain  Gain=1/Vdead2  ParameterDataType=sfix(16)  ParameterScaling=2^0  OutDataType=sfix(16)  OutScaling=2^0  SaturateOnIntegerOverflow=on
  Abs (v.t) : Abs  SaturateOnIntegerOverflow=on
  Integrator : Integrator  InitialCondition=Dead2CO2IC
  Product : Product  OutDataType=sfix(16)  OutScaling=2^0  SaturateOnIntegerOverflow=on  InputSameDT=on
  Sum : Sum  Inputs=-+  OutDataType=sfix(16)  OutScaling=2^0  SaturateOnIntegerOverflow=on  InputSameDT=on
  Switch : Switch  SaturateOnIntegerOverflow=on  InputSameDT=on
  Pd(2)CO2 : Outport  OutDataType=sfix(16)  OutScaling=2^0
  tag scope: Dead2CO2IC=global
  wires:
  Integrator/1 -> Pd(2)CO2/1, Sum/1, [Dead2CO2IC]
  Abs (v.t)/1 -> Product/2
  Flow/1 -> Abs (v.t)/1, Switch/2
  Pd(3)CO2/1 -> Switch/3
  Pd(1)CO2/1 -> Switch/1
  Sum/1 -> Product/1
  1/Vdead2/1 -> Integrator/1
  Product/1 -> 1/Vdead2/1
  Switch/1 -> Sum/2

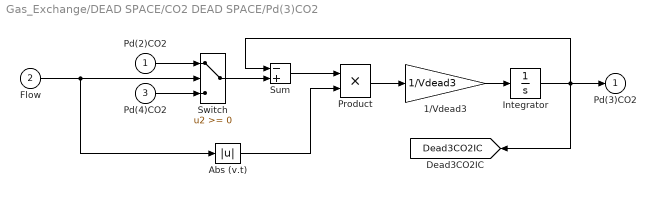
== system Gas_Exchange/DEAD SPACE/CO2 DEAD SPACE/Pd(3)CO2 ==
  Pd(2)CO2 : Inport  OutDataType=sfix(16)  OutScaling=2^0
  Flow : Inport  Port=2  OutDataType=sfix(16)  OutScaling=2^0
  Pd(4)CO2 : Inport  Port=3  OutDataType=sfix(16)  OutScaling=2^0
  1/Vdead3 : Gain  Gain=1/Vdead3  ParameterDataType=sfix(16)  ParameterScaling=2^0  OutDataType=sfix(16)  OutScaling=2^0  SaturateOnIntegerOverflow=on
  Abs (v.t) : Abs  SaturateOnIntegerOverflow=on
  Integrator : Integrator  InitialCondition=Dead3CO2IC
  Product : Product  OutDataType=sfix(16)  OutScaling=2^0  SaturateOnIntegerOverflow=on  InputSameDT=on
  Sum : Sum  Inputs=-+  OutDataType=sfix(16)  OutScaling=2^0  SaturateOnIntegerOverflow=on  InputSameDT=on
  Switch : Switch  SaturateOnIntegerOverflow=on  InputSameDT=on
  Pd(3)CO2 : Outport  OutDataType=sfix(16)  OutScaling=2^0
  tag scope: Dead3CO2IC=global
  wires:
  Abs (v.t)/1 -> Product/2
  Flow/1 -> Abs (v.t)/1, Switch/2
  Switch/1 -> Sum/2
  Product/1 -> 1/Vdead3/1
  1/Vdead3/1 -> Integrator/1
  Integrator/1 -> Sum/1, Pd(3)CO2/1, [Dead3CO2IC]
  Sum/1 -> Product/1
  Pd(2)CO2/1 -> Switch/1
  Pd(4)CO2/1 -> Switch/3

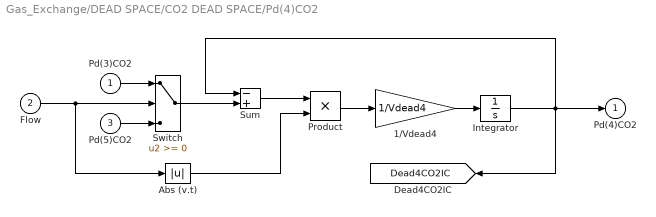
== system Gas_Exchange/DEAD SPACE/CO2 DEAD SPACE/Pd(4)CO2 ==
  Pd(3)CO2 : Inport  OutDataType=sfix(16)  OutScaling=2^0
  Flow : Inport  Port=2  OutDataType=sfix(16)  OutScaling=2^0
  Pd(5)CO2 : Inport  Port=3  OutDataType=sfix(16)  OutScaling=2^0
  1/Vdead4 : Gain  Gain=1/Vdead4  ParameterDataType=sfix(16)  ParameterScaling=2^0  OutDataType=sfix(16)  OutScaling=2^0  SaturateOnIntegerOverflow=on
  Abs (v.t) : Abs  SaturateOnIntegerOverflow=on
  Integrator : Integrator  InitialCondition=Dead4CO2IC
  Product : Product  OutDataType=sfix(16)  OutScaling=2^0  SaturateOnIntegerOverflow=on  InputSameDT=on
  Sum : Sum  Inputs=-+  OutDataType=sfix(16)  OutScaling=2^0  SaturateOnIntegerOverflow=on  InputSameDT=on
  Switch : Switch  SaturateOnIntegerOverflow=on  InputSameDT=on
  Pd(4)CO2 : Outport  OutDataType=sfix(16)  OutScaling=2^0
  tag scope: Dead4CO2IC=global
  wires:
  Abs (v.t)/1 -> Product/2
  Flow/1 -> Abs (v.t)/1, Switch/2
  Pd(5)CO2/1 -> Switch/3
  Pd(3)CO2/1 -> Switch/1
  Sum/1 -> Product/1
  1/Vdead4/1 -> Integrator/1
  Product/1 -> 1/Vdead4/1
  Switch/1 -> Sum/2
  Integrator/1 -> Pd(4)CO2/1, [Dead4CO2IC], Sum/1

== system Gas_Exchange/DEAD SPACE/CO2 DEAD SPACE/Pd(5)CO2 ==
  Pd(4)CO2 : Inport  OutDataType=sfix(16)  OutScaling=2^0
  Flow : Inport  Port=2  OutDataType=sfix(16)  OutScaling=2^0
  PACO2 : Inport  Port=3  OutDataType=sfix(16)  OutScaling=2^0
  1/Vdead5 : Gain  Gain=1/Vdead5  ParameterDataType=sfix(16)  ParameterScaling=2^0  OutDataType=sfix(16)  OutScaling=2^0  SaturateOnIntegerOverflow=on
  Abs (v.t) : Abs  SaturateOnIntegerOverflow=on
  Integrator : Integrator  InitialCondition=Dead5CO2IC
  Product : Product  OutDataType=sfix(16)  OutScaling=2^0  SaturateOnIntegerOverflow=on  InputSameDT=on
  Sum : Sum  Inputs=-+  OutDataType=sfix(16)  OutScaling=2^0  SaturateOnIntegerOverflow=on  InputSameDT=on
  Switch : Switch  SaturateOnIntegerOverflow=on  InputSameDT=on
  Pd(5)CO2 : Outport  OutDataType=sfix(16)  OutScaling=2^0
  tag scope: Dead5CO2IC=global
  wires:
  Abs (v.t)/1 -> Product/2
  Flow/1 -> Abs (v.t)/1, Switch/2
  Switch/1 -> Sum/2
  Product/1 -> 1/Vdead5/1
  1/Vdead5/1 -> Integrator/1
  Integrator/1 -> Sum/1, Pd(5)CO2/1, [Dead5CO2IC]
  Sum/1 -> Product/1
  Pd(4)CO2/1 -> Switch/1
  PACO2/1 -> Switch/3

== system Gas_Exchange/DEAD SPACE/O2 DEAD SPACE/O2 Partial Pressure ==
  Step : Step  Time=begin_time  Before=init_value  After=final_value  SampleTime=0
  Step1 : Step  Time=end_time  After=init_value-final_value  SampleTime=0
  Sum : Sum  Inputs=|++  OutDataType=sfix(16)  OutScaling=2^0  SaturateOnIntegerOverflow=on  InputSameDT=on
  Out1 : Outport  OutDataType=sfix(16)  OutScaling=2^0
  wires:
  Sum/1 -> Out1/1
  Step1/1 -> Sum/2
  Step/1 -> Sum/1

== system Gas_Exchange/DEAD SPACE/O2 DEAD SPACE/Pd(1)O2 ==
  PIO2 : Inport  OutDataType=sfix(16)  OutScaling=2^0
  Flow : Inport  Port=2  OutDataType=sfix(16)  OutScaling=2^0
  Pd(2)O2 : Inport  Port=3  OutDataType=sfix(16)  OutScaling=2^0
  1/Vdead1 : Gain  Gain=1/Vdead1  ParameterDataType=sfix(16)  ParameterScaling=2^0  OutDataType=sfix(16)  OutScaling=2^0  SaturateOnIntegerOverflow=on
  Abs (v.t) : Abs  SaturateOnIntegerOverflow=on
  Integrator : Integrator  InitialCondition=Dead1O2IC
  Product : Product  OutDataType=sfix(16)  OutScaling=2^0  SaturateOnIntegerOverflow=on  InputSameDT=on
  Sum : Sum  Inputs=-+  OutDataType=sfix(16)  OutScaling=2^0  SaturateOnIntegerOverflow=on  InputSameDT=on
  Switch : Switch  SaturateOnIntegerOverflow=on  InputSameDT=on
  Pd(1)O2 : Outport  OutDataType=sfix(16)  OutScaling=2^0
  tag scope: Dead1O2IC=global
  wires:
  Switch/1 -> Sum/2
  Pd(2)O2/1 -> Switch/3
  PIO2/1 -> Switch/1
  Sum/1 -> Product/1
  Integrator/1 -> Sum/1, Pd(1)O2/1, [Dead1O2IC]
  1/Vdead1/1 -> Integrator/1
  Product/1 -> 1/Vdead1/1
  Flow/1 -> Abs (v.t)/1, Switch/2
  Abs (v.t)/1 -> Product/2

== system Gas_Exchange/DEAD SPACE/O2 DEAD SPACE/Pd(2)O2 ==
  Pd(1)O2 : Inport  OutDataType=sfix(16)  OutScaling=2^0
  Flow : Inport  Port=2  OutDataType=sfix(16)  OutScaling=2^0
  Pd(3)O2 : Inport  Port=3  OutDataType=sfix(16)  OutScaling=2^0
  1/Vdead2 : Gain  Gain=1/Vdead2  ParameterDataType=sfix(16)  ParameterScaling=2^0  OutDataType=sfix(16)  OutScaling=2^0  SaturateOnIntegerOverflow=on
  Abs (v.t) : Abs  SaturateOnIntegerOverflow=on
  Integrator : Integrator  InitialCondition=Dead2O2IC
  Product : Product  OutDataType=sfix(16)  OutScaling=2^0  SaturateOnIntegerOverflow=on  InputSameDT=on
  Sum : Sum  Inputs=-+  OutDataType=sfix(16)  OutScaling=2^0  SaturateOnIntegerOverflow=on  InputSameDT=on
  Switch : Switch  SaturateOnIntegerOverflow=on  InputSameDT=on
  Pd(2)O2 : Outport  OutDataType=sfix(16)  OutScaling=2^0
  tag scope: Dead2O2IC=global
  wires:
  Abs (v.t)/1 -> Product/2
  Flow/1 -> Abs (v.t)/1, Switch/2
  Product/1 -> 1/Vdead2/1
  Integrator/1 -> [Dead2O2IC], Sum/1, Pd(2)O2/1
  Sum/1 -> Product/1
  Pd(1)O2/1 -> Switch/1
  Pd(3)O2/1 -> Switch/3
  Switch/1 -> Sum/2
  1/Vdead2/1 -> Integrator/1

== system Gas_Exchange/DEAD SPACE/O2 DEAD SPACE/Pd(3)O2 ==
  Pd(2)O2 : Inport  OutDataType=sfix(16)  OutScaling=2^0
  Flow : Inport  Port=2  OutDataType=sfix(16)  OutScaling=2^0
  Pd(4)O2 : Inport  Port=3  OutDataType=sfix(16)  OutScaling=2^0
  1/Vdead3 : Gain  Gain=1/Vdead3  ParameterDataType=sfix(16)  ParameterScaling=2^0  OutDataType=sfix(16)  OutScaling=2^0  SaturateOnIntegerOverflow=on
  Abs (v.t) : Abs  SaturateOnIntegerOverflow=on
  Integrator : Integrator  InitialCondition=Dead3O2IC
  Product : Product  OutDataType=sfix(16)  OutScaling=2^0  SaturateOnIntegerOverflow=on  InputSameDT=on
  Sum : Sum  Inputs=-+  OutDataType=sfix(16)  OutScaling=2^0  SaturateOnIntegerOverflow=on  InputSameDT=on
  Switch : Switch  SaturateOnIntegerOverflow=on  InputSameDT=on
  Pd(3)O2 : Outport  OutDataType=sfix(16)  OutScaling=2^0
  tag scope: Dead3O2IC=global
  wires:
  Switch/1 -> Sum/2
  Pd(4)O2/1 -> Switch/3
  Pd(2)O2/1 -> Switch/1
  Sum/1 -> Product/1
  Integrator/1 -> [Dead3O2IC], Sum/1, Pd(3)O2/1
  Product/1 -> 1/Vdead3/1
  Flow/1 -> Abs (v.t)/1, Switch/2
  Abs (v.t)/1 -> Product/2
  1/Vdead3/1 -> Integrator/1

== system Gas_Exchange/DEAD SPACE/O2 DEAD SPACE/Pd(4)O2 ==
  Pd(3)O2 : Inport  OutDataType=sfix(16)  OutScaling=2^0
  Flow : Inport  Port=2  OutDataType=sfix(16)  OutScaling=2^0
  Pd(5)O2 : Inport  Port=3  OutDataType=sfix(16)  OutScaling=2^0
  1/Vdead4 : Gain  Gain=1/Vdead4  ParameterDataType=sfix(16)  ParameterScaling=2^0  OutDataType=sfix(16)  OutScaling=2^0  SaturateOnIntegerOverflow=on
  Abs (v.t) : Abs  SaturateOnIntegerOverflow=on
  Integrator : Integrator  InitialCondition=Dead4O2IC
  Product : Product  OutDataType=sfix(16)  OutScaling=2^0  SaturateOnIntegerOverflow=on  InputSameDT=on
  Sum : Sum  Inputs=-+  OutDataType=sfix(16)  OutScaling=2^0  SaturateOnIntegerOverflow=on  InputSameDT=on
  Switch : Switch  SaturateOnIntegerOverflow=on  InputSameDT=on
  Pd(4)O2 : Outport  OutDataType=sfix(16)  OutScaling=2^0
  tag scope: Dead4O2IC=global
  wires:
  Abs (v.t)/1 -> Product/2
  Flow/1 -> Abs (v.t)/1, Switch/2
  Product/1 -> 1/Vdead4/1
  Integrator/1 -> Sum/1, Pd(4)O2/1, [Dead4O2IC]
  Sum/1 -> Product/1
  Pd(3)O2/1 -> Switch/1
  Pd(5)O2/1 -> Switch/3
  Switch/1 -> Sum/2
  1/Vdead4/1 -> Integrator/1

== system Gas_Exchange/DEAD SPACE/O2 DEAD SPACE/Pd(5)O2 ==
  Pd(4)O2 : Inport  OutDataType=sfix(16)  OutScaling=2^0
  Flow : Inport  Port=2  OutDataType=sfix(16)  OutScaling=2^0
  PAO2 : Inport  Port=3  OutDataType=sfix(16)  OutScaling=2^0
  1/Vdead5 : Gain  Gain=1/Vdead5  ParameterDataType=sfix(16)  ParameterScaling=2^0  OutDataType=sfix(16)  OutScaling=2^0  SaturateOnIntegerOverflow=on
  Abs (v.t) : Abs  SaturateOnIntegerOverflow=on
  Integrator : Integrator  InitialCondition=Dead5O2IC
  Product : Product  OutDataType=sfix(16)  OutScaling=2^0  SaturateOnIntegerOverflow=on  InputSameDT=on
  Sum : Sum  Inputs=-+  OutDataType=sfix(16)  OutScaling=2^0  SaturateOnIntegerOverflow=on  InputSameDT=on
  Switch : Switch  SaturateOnIntegerOverflow=on  InputSameDT=on
  Pd(5)O2 : Outport  OutDataType=sfix(16)  OutScaling=2^0
  tag scope: Dead5O2IC=global
  wires:
  Switch/1 -> Sum/2
  PAO2/1 -> Switch/3
  Pd(4)O2/1 -> Switch/1
  Sum/1 -> Product/1
  Integrator/1 -> Pd(5)O2/1, [Dead5O2IC], Sum/1
  Product/1 -> 1/Vdead5/1
  Flow/1 -> Abs (v.t)/1, Switch/2
  Abs (v.t)/1 -> Product/2
  1/Vdead5/1 -> Integrator/1

== system Gas_Exchange/DEAD SPACE/CO2 DEAD SPACE/CO2 Partial Pressure/If Action Subsystem ==
  In1 : Inport  OutDataType=sfix(16)  OutScaling=2^0
  In2 : Inport  Port=2  OutDataType=sfix(16)  OutScaling=2^0
  Action Port : ActionPort
  Integrator : Integrator
  Product1 : Product  OutDataType=sfix(16)  OutScaling=2^0  RndMeth=Zero
  Out1 : Outport  OutDataType=sfix(16)  OutScaling=2^0  InitialOutput=0
  wires:
  Product1/1 -> Integrator/1
  In2/1 -> Product1/2
  In1/1 -> Product1/1
  Integrator/1 -> Out1/1

== system Gas_Exchange/DEAD SPACE/CO2 DEAD SPACE/CO2 Partial Pressure/If Action Subsystem1 ==
  In1 : Inport  OutDataType=sfix(16)  OutScaling=2^0
  In2 : Inport  Port=2  OutDataType=sfix(16)  OutScaling=2^0
  Action Port : ActionPort
  Integrator : Integrator
  Product1 : Product  OutDataType=sfix(16)  OutScaling=2^0  RndMeth=Zero
  Out1 : Outport  OutDataType=sfix(16)  OutScaling=2^0  InitialOutput=0
  wires:
  Product1/1 -> Integrator/1
  In2/1 -> Product1/2
  In1/1 -> Product1/1
  Integrator/1 -> Out1/1
